simulink model "simulinkQ1c"  (R2022a)
settings: Solver=VariableStepAuto  StartTime=0.0  StopTime=10.0  RelTol=1e-3
settings Model: Creator=ABHIJIT NIT  LastModifiedBy=heera
settings DebuggingCC: UnconnectedInputMsg=warning  UnconnectedOutputMsg=warning  UnconnectedLineMsg=warning
settings RTWCC: DLArmComputeVersion=19.05

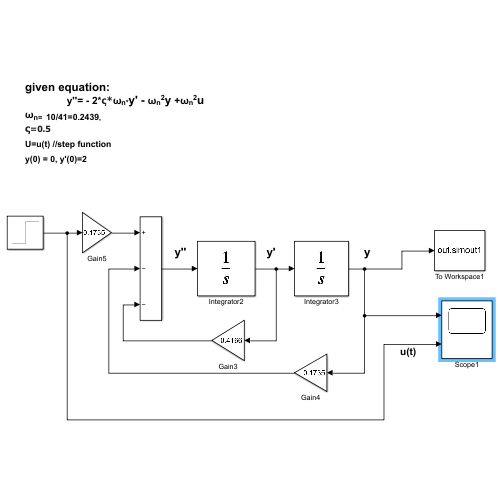
[thumbnail: Simulink's stored preview of the top-level diagram]
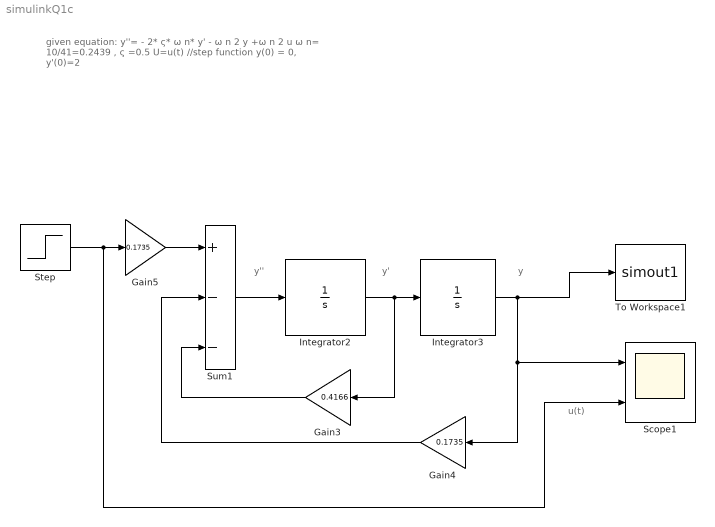
== system simulinkQ1c ==
  note: u(t)
  note: y
  note: y'
  note: y''
  note: given equation:
      | y''= - 2* ς* ω n* y' - ω n 2 y +ω n 2 u
      | ω n= 10/41=0.2439 ,
      | ς =0.5
      | U=u(t) //step function
      | y(0) = 0, y'(0)=2
  Gain3 : Gain  Gain=0.4166
  Gain4 : Gain  Gain=0.1735
  Gain5 : Gain  Gain=0.1735
  Integrator2 : Integrator  InitialCondition=2
  Integrator3 : Integrator
  Scope1 : Scope  NumInputPorts=2
  Step : Step  SampleTime=0
  Sum1 : Sum  Inputs=+--
  To Workspace1 : ToWorkspace  VariableName=simout1  SaveFormat=Timeseries  SampleTime=-1
  wires:
  Step/1 -> Gain5/1, Scope1/2
  Integrator3/1 -> Gain4/1, Scope1/1, To Workspace1/1
  Gain5/1 -> Sum1/1
  Gain3/1 -> Sum1/3
  Gain4/1 -> Sum1/2
  Sum1/1 -> Integrator2/1
  Integrator2/1 -> Gain3/1, Integrator3/1
